simulink model "HILModel_flightgear"  (Simulink 7.8)
settings: Solver=ode4  StartTime=0.0  StopTime=inf  FixedStep=SampleT  RelTol=1e-3
InitFcn:
  | clc
  | hilInit
  | launchFlightgear
values from neighbouring files (symbols this model uses):
  Euler_0 = [0; 0*pi/180; 0*pi/180]'    [hilInit.m]
  HIL_K = 3    [hilInit.m]
  Pos_0 = [0; 0; 150]'    [hilInit.m]
  SampleT = 0.005    [hilInit.m]
  Vb_0 = [ 17; 0; 0]'    [hilInit.m]
  windBase = 3.5    [hilInit.m]
undefined symbols (not defined in the file or in its folder): A1, Apolar, barAdjust, baroOffset, baroScale, barTGain2, barTMean2, bPWMda, bPWMde, bPWMdr, bPWMdt, CD0, chord, CL0, CLa, CLa_dot, Clb, ClDa, CLDe, CLDf, ClDr, clock, Clp, CLq, Clr, Cm0, Cma, CmDe, CmDf, Cmq, Cnb, CnDa, CnDr, Cnp, Cnr, cubeAccelGain16405, cubeGyroGain16405, cubeMagGain16405, CYb, CYDr, da_failamp, da_failbias, da_failper, daL_fail, daR_fail, DiscIntNeverNeededParam, dr_fail, Earth, elarm, F, GS_location, ISA_g, Ixx, Iyy, Izz, Light, mass, MIL, MinThK, mPWMda ... (+14)
libraries: simulink x30, aerolibconvert2 x11, xpclib x8, aerolibactuator x5, aerolibwind2 x2, dspmtrx3 x2, aerolibfltsims x2, aerolibtransform2 x1, aerolibobsolete x1, aerolibatmos2 x1, aerolibanimutils x1
(part 1 of 3)
CloseFcn:
  | rtwprivate ssgencode ModelCloseRequest AttitudeComplementary
settings Model: Creator=ASL_Lab  LastModifiedBy=dagoodma
settings OptimizationCC: InitFltsAndDblsToZero=on
settings DebuggingCC: AlgebraicLoopMsg=error  SaveWithParameterizedLinksMsg=none  MultiTaskDSMMsg=warning  MultiTaskCondExecSysMsg=none  FcnCallInpInsideContextMsg=Use local settings  StrictBusMsg=None
settings HardwareCC: TargetHWDeviceType=32-bit Generic
settings SFSimCC: SimParseCustomCode=off
settings RTWCC: IncludeERTFirstTime=on
settings GRTTargetCC: TargetFcnLib=ansi_tfl_tmw.mat

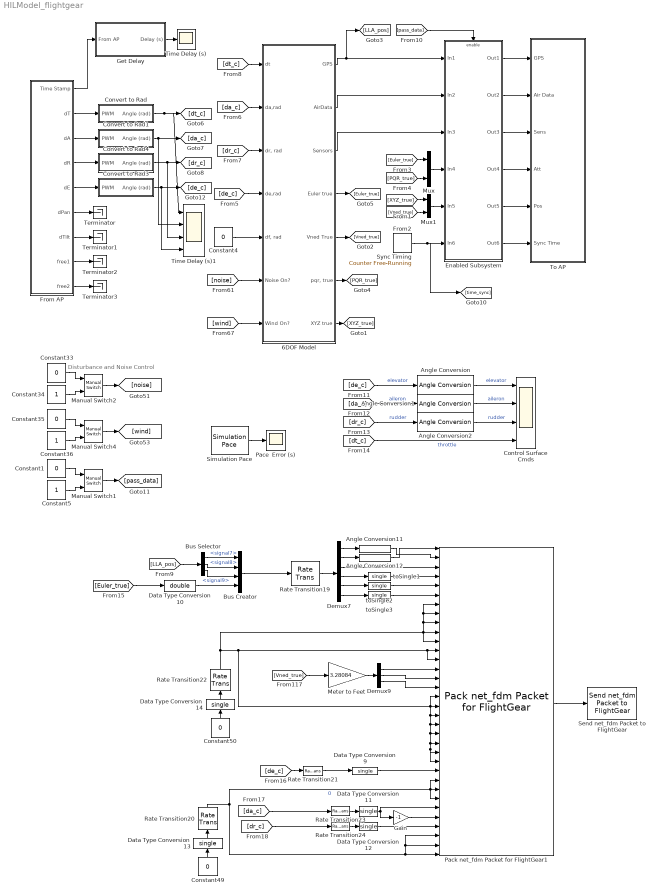
== system HILModel_flightgear ==
  note: Disturbance and Noise Control
  6DOF Model : Subsystem
  Angle Conversion : aerolibconvert2/Angle Conversion  IU=rad  OU=deg
  Angle Conversion1 : aerolibconvert2/Angle Conversion  IU=rad  OU=deg
  Angle Conversion11 : aerolibconvert2/Angle Conversion  IU=deg  OU=rad
  Angle Conversion12 : aerolibconvert2/Angle Conversion  IU=deg  OU=rad
  Angle Conversion2 : aerolibconvert2/Angle Conversion  IU=rad  OU=deg
  Bus Creator : BusCreator
  Bus Selector : BusSelector  OutputSignals=signal7,signal8,signal9
  Constant1 : Constant  Value=0  SampleTime=SampleT
  Constant33 : Constant  Value=0  SampleTime=SampleT
  Constant34 : Constant  SampleTime=SampleT
  Constant35 : Constant  Value=0  SampleTime=SampleT
  Constant36 : Constant  SampleTime=SampleT
  Constant4 : Constant  Value=0
  Constant49 : Constant  Value=0
  Constant5 : Constant  SampleTime=SampleT
  Constant50 : Constant  Value=0
  Control Surface Cmds : Scope  NumInputPorts=4
      settings: TimeRange=70  YMin=0.475~1.425~1.44~0.05  YMax=0.545~1.65~1.57~0.55  MaxDataPoints=25000
  Convert to Rad : Subsystem  mask{slopem=mPWMdt, interceptb=bPWMdt}
      mask prompts: slopem "Slope"; interceptb "Intercept"
  Convert to Rad1 : Subsystem  mask{slopem=mPWMda, interceptb=bPWMda}
      mask prompts: slopem "Slope"; interceptb "Intercept"
  Convert to Rad3 : Subsystem  mask{slopem=mPWMde, interceptb=bPWMde}
      mask prompts: slopem "Slope"; interceptb "Intercept"
  Convert to Rad4 : Subsystem  mask{slopem=mPWMdr, interceptb=bPWMdr}
      mask prompts: slopem "Slope"; interceptb "Intercept"
  Data Type Conversion10 : DataTypeConversion  OutDataTypeStr=double
  Data Type Conversion{9,11..14} (5 alike) : DataTypeConversion  OutDataTypeStr=single
  Demux7 : Demux  Outputs=6
  Demux9 : Demux  Outputs=3
  Enabled Subsystem : Subsystem  TreatAsAtomicUnit=on
  From AP : Subsystem
  Gain : Gain  Gain=-1
  Get Delay : Subsystem
  Manual Switch1 : simulink/Signal Routing/Manual Switch  sw=0  action=0  varsize=off
  Manual Switch2 : simulink/Signal Routing/Manual Switch  sw=1  action=0  varsize=off
  Manual Switch4 : simulink/Signal Routing/Manual Switch  sw=1  action=0  varsize=off
  Meter to Feet : Gain  Gain=3.28084
  Mux : Mux  Inputs=2
  Mux1 : Mux  Inputs=2
  Pace  Error (s) : Scope
      settings: YMin=-0.01  YMax=0.015  MaxDataPoints=25000
  Pack net_fdm Packet for FlightGear1 : aerolibfltsims/Pack net_fdm Packet for FlightGear  FlightGearVersion=v2.0  ShowPositionAttitudeInputs=on  ShowVelocityAccelerationInputs=on  ShowControlSurfacePositionInputs=on  ShowEngineFuelInputs=off  ShowLandingGearInputs=off  ShowEnvironmentInputs=off  SampleTime=SampleT
  Rate Transition{19,21,23..24} (4 alike) : RateTransition  Integrity=off  Deterministic=off  OutPortSampleTime=SampleT
  Rate Transition20 : RateTransition  OutPortSampleTime=SampleT
  Rate Transition22 : RateTransition  OutPortSampleTime=SampleT
  Send net_fdm Packet to FlightGear : aerolibfltsims/Send net_fdm Packet to FlightGear  DestinationIpAddress=127.0.0.1  DestinationPort=FLIGHTGEAR_UDP_FDM_PORT  LocalIpPort=-1  varLen=off  SampleTime=SampleT
  Simulation Pace : aerolibanimutils/Simulation Pace  SimulationPace=1  SleepMode=MATLAB Thread  OutputPaceError=on  SampleTime=SampleT
      settings: AttributesFormatString=%<SimulationPace> sec/sec
  Sync Timing : simulink/Sources/Counter Free-Running  NumBits=32  tsamp=SampleT
  Terminator{,1..3} (4 alike) : Terminator
  Time Delay (s) : Scope
      settings: TimeRange=60  YMin=0  YMax=0.05  SaveName=ScopeData2
  Time Delay (s)1 : Scope  NumInputPorts=4
      settings: TimeRange=60  YMin=-2.49294~0.78707~1.28363~-0.624215  YMax=-2.49294~0.78707~1.28363~-0.624215  SaveName=ScopeData3
  To AP : Subsystem
  toSingle1 : DataTypeConversion  OutDataTypeStr=single
  toSingle2 : DataTypeConversion  OutDataTypeStr=single
  toSingle3 : DataTypeConversion  OutDataTypeStr=single
  wires:
  [PQR_true] -> Mux/2
  [XYZ_true] -> Mux1/1
  [Vned_true] -> Mux1/2
  [Euler_true] -> Mux/1
  Enabled Subsystem/1(Out1) -> To AP/1(GPS)
  Enabled Subsystem/2(Out2) -> To AP/2(Air Data)
  Enabled Subsystem/3(Out3) -> To AP/3(Sens)
  Enabled Subsystem/4(Out4) -> To AP/4(Att)
  Enabled Subsystem/5(Out5) -> To AP/5(Pos)
  Enabled Subsystem/6(Out6) -> To AP/6(Sync Time)
  6DOF Model/1(GPS) -> Enabled Subsystem/1(In1), [LLA_pos]
  6DOF Model/2(AirData) -> Enabled Subsystem/2(In2)
  6DOF Model/3(Sensors) -> Enabled Subsystem/3(In3)
  Mux/1 -> Enabled Subsystem/4(In4)
  Mux1/1 -> Enabled Subsystem/5(In5)
  Sync Timing/1 -> Enabled Subsystem/6(In6), [time_sync]
  6DOF Model/4(Euler true) -> [Euler_true]
  6DOF Model/5(Vned True) -> [Vned_true]
  6DOF Model/6("pqr, true") -> [PQR_true]
  6DOF Model/7(XYZ true) -> [XYZ_true]
  Constant4/1 -> 6DOF Model/5("df, rad")
  Constant33/1 -> Manual Switch2/1
  Constant34/1 -> Manual Switch2/2
  Manual Switch2/1 -> [noise]
  Constant35/1 -> Manual Switch4/1
  Constant36/1 -> Manual Switch4/2
  Manual Switch4/1 -> [wind]
  [noise] -> 6DOF Model/6(Noise On?)
  [wind] -> 6DOF Model/7(Wind On?)
  Constant1/1 -> Manual Switch1/1
  Constant5/1 -> Manual Switch1/2
  Manual Switch1/1 -> [pass_data]
  [pass_data] -> Enabled Subsystem/Enable
  From AP/3(dA) -> Convert to Rad1/1(PWM)
  From AP/5(dE) -> Convert to Rad3/1(PWM)
  From AP/2(dT) -> Convert to Rad/1(PWM)
  From AP/4(dR) -> Convert to Rad4/1(PWM)
  Get Delay/1(Delay (s)) -> Time Delay (s)/1
  From AP/1(Time Stamp) -> Get Delay/1(From AP)
  Convert to Rad/1(Angle (rad)) -> [dt_c], Time Delay (s)1/1
  Convert to Rad1/1(Angle (rad)) -> [da_c], Time Delay (s)1/2
  From AP/6(dPan) -> Terminator/1
  [de_c] -> Angle Conversion/1  "elevator"
  [da_c] -> Angle Conversion1/1  "aileron"
  [dr_c] -> Angle Conversion2/1  "rudder"
  [dt_c] -> Control Surface Cmds/4  "throttle"
  [de_c] -> 6DOF Model/4(de,rad)
  [dt_c] -> 6DOF Model/1(dt)
  [dr_c] -> 6DOF Model/3("dr, rad")
  [da_c] -> 6DOF Model/2(da,rad)
  Angle Conversion/1 -> Control Surface Cmds/1  "elevator"
  Angle Conversion1/1 -> Control Surface Cmds/2  "aileron"
  Angle Conversion2/1 -> Control Surface Cmds/3  "rudder"
  Simulation Pace/1 -> Pace  Error (s)/1
  Convert to Rad4/1(Angle (rad)) -> [dr_c], Time Delay (s)1/3
  Convert to Rad3/1(Angle (rad)) -> [de_c], Time Delay (s)1/4
  From AP/7(dTilt) -> Terminator1/1
  From AP/8(free1) -> Terminator2/1
  From AP/9(free2) -> Terminator3/1
  Rate Transition19/1 -> Demux7/1
  Demux7/1 -> Angle Conversion11/1
  Demux7/2 -> Angle Conversion12/1
  Demux7/3 -> Pack net_fdm Packet for FlightGear1/3
  Demux7/4 -> toSingle1/1
  Demux7/5 -> toSingle2/1
  Demux7/6 -> toSingle3/1
  toSingle1/1 -> Pack net_fdm Packet for FlightGear1/4
  toSingle2/1 -> Pack net_fdm Packet for FlightGear1/5
  toSingle3/1 -> Pack net_fdm Packet for FlightGear1/6
  Pack net_fdm Packet for FlightGear1/1 -> Send net_fdm Packet to FlightGear/1
  Data Type Conversion12/1 -> Pack net_fdm Packet for FlightGear1/31
  Rate Transition20/1 -> Pack net_fdm Packet for FlightGear1/34, Pack net_fdm Packet for FlightGear1/33, Pack net_fdm Packet for FlightGear1/32, Pack net_fdm Packet for FlightGear1/26, Pack net_fdm Packet for FlightGear1/27, Pack net_fdm Packet for FlightGear1/28  "0"
  Rate Transition21/1 -> Data Type Conversion9/1
  Rate Transition23/1 -> Data Type Conversion11/1
  Data Type Conversion13/1 -> Rate Transition20/1
  Constant49/1 -> Data Type Conversion13/1
  Rate Transition24/1 -> Data Type Conversion12/1
  Data Type Conversion11/1 -> Gain/1, Pack net_fdm Packet for FlightGear1/29
  Gain/1 -> Pack net_fdm Packet for FlightGear1/30
  Angle Conversion12/1 -> Pack net_fdm Packet for FlightGear1/1
  Angle Conversion11/1 -> Pack net_fdm Packet for FlightGear1/2
  Data Type Conversion9/1 -> Pack net_fdm Packet for FlightGear1/25
  Data Type Conversion14/1 -> Rate Transition22/1
  Constant50/1 -> Data Type Conversion14/1
  Rate Transition22/1 -> Pack net_fdm Packet for FlightGear1/10, Pack net_fdm Packet for FlightGear1/11, Pack net_fdm Packet for FlightGear1/9, Pack net_fdm Packet for FlightGear1/7, Pack net_fdm Packet for FlightGear1/8, Pack net_fdm Packet for FlightGear1/12, Pack net_fdm Packet for FlightGear1/13, Pack net_fdm Packet for FlightGear1/18, Pack net_fdm Packet for FlightGear1/17, Pack net_fdm Packet for FlightGear1/19, Pack net_fdm Packet for FlightGear1/20, Pack net_fdm Packet for FlightGear1/21, Pack net_fdm Packet for FlightGear1/22, Pack net_fdm Packet for FlightGear1/23, Pack net_fdm Packet for FlightGear1/24
  Demux9/1 -> Pack net_fdm Packet for FlightGear1/14
  Demux9/3 -> Pack net_fdm Packet for FlightGear1/16
  Demux9/2 -> Pack net_fdm Packet for FlightGear1/15
  [Vned_true] -> Meter to Feet/1
  Meter to Feet/1 -> Demux9/1
  [Euler_true] -> Data Type Conversion10/1
  [LLA_pos] -> Bus Selector/1
  Bus Selector/1 -> Bus Creator/1  "<signal7>"
  Bus Selector/2 -> Bus Creator/2  "<signal8>"
  Bus Selector/3 -> Bus Creator/3  "<signal9>"
  Data Type Conversion10/1 -> Bus Creator/4
  Bus Creator/1 -> Rate Transition19/1
  [de_c] -> Rate Transition21/1
  [da_c] -> Rate Transition23/1
  [dr_c] -> Rate Transition24/1

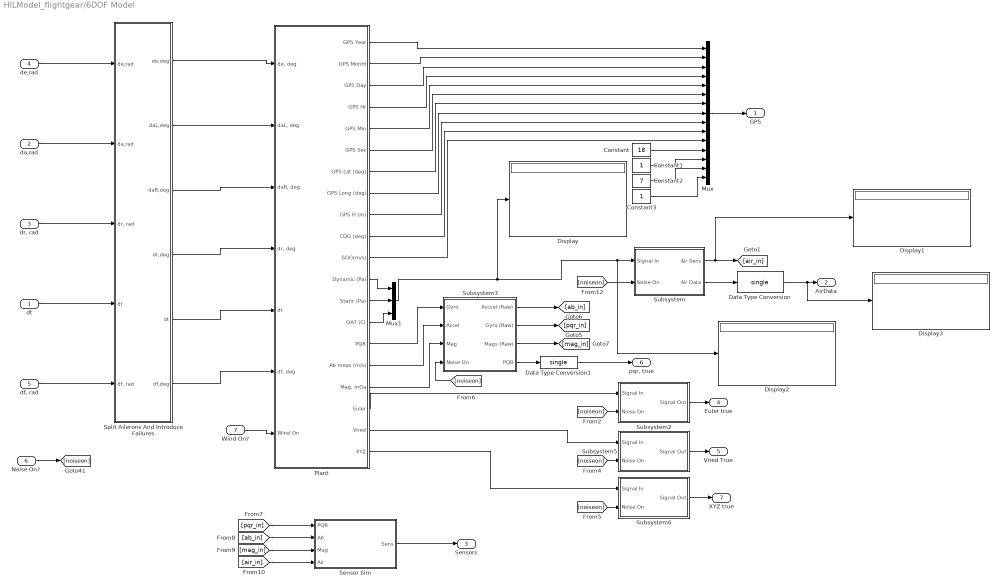
== system HILModel_flightgear/6DOF Model ==
  dt : Inport
  da,rad : Inport  Port=2
  "dr, rad" : Inport  Port=3
  de,rad : Inport  Port=4
  "df, rad" : Inport  Port=5
  Noise On? : Inport  Port=6
  Wind On? : Inport  Port=7
  Constant : Constant  Value=18  SampleTime=SampleT
  Constant1 : Constant  SampleTime=SampleT
  Constant2 : Constant  Value=7  SampleTime=SampleT
  Constant3 : Constant  SampleTime=SampleT
  Data Type Conversion : DataTypeConversion  OutDataTypeStr=single
  Data Type Conversion1 : DataTypeConversion  OutDataTypeStr=single
  Display{,1..3} (4 alike) : Display
  Mux : Mux  Inputs=15
  Mux1 : Mux  Inputs=3
  Plant : Subsystem
  Sensor Sim : Subsystem
  Split Ailerons And Introduce Failures : Subsystem
  Subsystem : Subsystem  mask{nv=[0.01 0.01 0.1], st=SampleT, ns=[132 564 987]}
      mask prompts: nv "Noise Variance"; st "Sample Time"; ns "Noise Seed"
  Subsystem2 : Subsystem  mask{nv=[0.0001 0.00003 0.0001], st=SampleT, ns=[132 564 987]}
      mask prompts: nv "Noise Variance"; st "Sample Time"; ns "Noise Seed"
  Subsystem3 : Subsystem  mask{accelVar=[0.1 0.1 0.1], accelSeed=[132 564 987], hilCubeAccelGain=cubeAccelGain16405, gyroVar=[0.1 0.1 0.1], gyroSeed=[132 564 987], hilCubeGyroGain=cubeGyroGain16405, magVar=[0.1 0.1 0.1], magSeed=[132 564 987], hilCubeMagGain=cubeMagGain16405, st=SampleT}
      mask prompts: accelVar "Accelerometer Noise Variance"; accelSeed "Accelerometer Noise Seed"; hilCubeAccelGain "Accelerometer Gain"; gyroVar "Gyro Noise Variance"; gyroSeed "Gyro Noise Seed"; hilCubeGyroGain "Gyro Gain"; magVar "Magnetometer Noise Variance"; magSeed "Magnetometer Noise Seed"; hilCubeMagGain "Magnetometer Gain"; st "Sample Time"
  Subsystem5 : Subsystem  mask{nv=[0.01 0.01 0.01], st=SampleT, ns=[321564 6546 98798]}
      mask prompts: nv "Noise Variance"; st "Sample Time"; ns "Noise Seed"
  Subsystem6 : Subsystem  mask{nv=[0.05 0.05 0.07], st=SampleT, ns=[321564]}
      mask prompts: nv "Noise Variance"; st "Sample Time"; ns "Noise Seed"
  GPS : Outport
  AirData : Outport  Port=2
  Sensors : Outport  Port=3
  Euler true : Outport  Port=4
  Vned True : Outport  Port=5
  "pqr, true" : Outport  Port=6
  XYZ true : Outport  Port=7
  wires:
  Data Type Conversion/1 -> AirData/1, Display3/1
  Wind On?/1 -> Plant/7(Wind On)
  Plant/20(XYZ) -> Subsystem6/1(Signal In)
  Subsystem6/1(Signal Out) -> XYZ true/1
  Plant/19(Vned) -> Subsystem5/1(Signal In)
  Subsystem5/1(Signal Out) -> Vned True/1
  Plant/18(Euler) -> Subsystem2/1(Signal In)
  Subsystem2/1(Signal Out) -> Euler true/1
  [noiseon] -> Subsystem3/4(Noise On)
  [noiseon] -> Subsystem6/2(Noise On)
  [noiseon] -> Subsystem5/2(Noise On)
  [noiseon] -> Subsystem2/2(Noise On)
  [noiseon] -> Subsystem/2(Noise On)
  Subsystem/1(Air Sens) -> [air_in], Display1/1
  Noise On?/1 -> [noiseon]
  Constant3/1 -> Mux/15
  Constant2/1 -> Mux/14
  Constant1/1 -> Mux/13
  Constant/1 -> Mux/12
  Mux1/1 -> Subsystem/1(Signal In), Display2/1, Display/1
  Plant/14(OAT (C)) -> Mux1/3
  Plant/13(Static (Pa)) -> Mux1/2
  Plant/11(SOG(m/s)) -> Mux/11
  Plant/10(COG (deg)) -> Mux/10
  Plant/9(GPS H (m)) -> Mux/9
  Plant/8(GPS Long (deg)) -> Mux/8
  Plant/7(GPS Lat (deg)) -> Mux/7
  Plant/6(GPS Sec) -> Mux/6
  Plant/5(GPS Min) -> Mux/5
  Plant/4(GPS Hr) -> Mux/4
  Plant/3(GPS Day) -> Mux/3
  Plant/2(GPS Month) -> Mux/2
  Plant/1(GPS Year) -> Mux/1
  Mux/1 -> GPS/1
  "df, rad"/1 -> Split Ailerons And Introduce Failures/5("df, rad")
  dt/1 -> Split Ailerons And Introduce Failures/4(dt)
  "dr, rad"/1 -> Split Ailerons And Introduce Failures/3("dr, rad")
  da,rad/1 -> Split Ailerons And Introduce Failures/2(da,rad)
  de,rad/1 -> Split Ailerons And Introduce Failures/1(de,rad)
  [pqr_in] -> Sensor Sim/1(PQR)
  [ab_in] -> Sensor Sim/2(Ab)
  [mag_in] -> Sensor Sim/3(Mag)
  Split Ailerons And Introduce Failures/1(de,deg) -> Plant/1("de, deg")
  Split Ailerons And Introduce Failures/2(daL,deg) -> Plant/2("daL, deg")
  Split Ailerons And Introduce Failures/3(daR,deg) -> Plant/3("daR, deg")
  Split Ailerons And Introduce Failures/4(dr,deg) -> Plant/4("dr, deg")
  Split Ailerons And Introduce Failures/5("dt ") -> Plant/5(dt)
  Split Ailerons And Introduce Failures/6(df,deg) -> Plant/6("df, deg")
  [air_in] -> Sensor Sim/4(Air)
  Plant/15(PQR) -> Subsystem3/1(Gyro)
  Plant/16(Ab meas (m/s)) -> Subsystem3/2(Accel)
  Plant/17("Mag, mGa") -> Subsystem3/3(Mag)
  Subsystem3/4("PQR ") -> Data Type Conversion1/1
  Subsystem3/1(Acccel (Raw)) -> [ab_in]
  Subsystem3/2("Gyro (Raw)  ") -> [pqr_in]
  Subsystem3/3(Mags (Raw)) -> [mag_in]
  Sensor Sim/1(Sens) -> Sensors/1
  Data Type Conversion1/1 -> "pqr, true"/1
  Subsystem/2(Air Data) -> Data Type Conversion/1
  Plant/12(Dynamic (Pa)) -> Mux1/1

== system HILModel_flightgear/Convert to Rad ==
  PWM : Inport
  Add : Sum
  Constant1 : Constant  Value=slopem
  Constant2 : Constant  Value=interceptb
  Data Type Conversion : DataTypeConversion  OutDataTypeStr=single
  Divide : Product
  Angle (rad) : Outport
  wires:
  Constant1/1 -> Divide/2
  Add/1 -> Data Type Conversion/1
  Divide/1 -> Add/1
  Constant2/1 -> Add/2
  PWM/1 -> Divide/1
  Data Type Conversion/1 -> Angle (rad)/1

== system HILModel_flightgear/Convert to Rad1 ==
  PWM : Inport
  Add : Sum
  Constant1 : Constant  Value=slopem
  Constant2 : Constant  Value=interceptb
  Data Type Conversion : DataTypeConversion  OutDataTypeStr=single
  Divide : Product
  Angle (rad) : Outport
  wires:
  Data Type Conversion/1 -> Angle (rad)/1
  PWM/1 -> Divide/1
  Constant2/1 -> Add/2
  Divide/1 -> Add/1
  Add/1 -> Data Type Conversion/1
  Constant1/1 -> Divide/2

== system HILModel_flightgear/Convert to Rad3 ==
  PWM : Inport
  Add : Sum
  Constant1 : Constant  Value=slopem
  Constant2 : Constant  Value=interceptb
  Data Type Conversion : DataTypeConversion  OutDataTypeStr=single
  Divide : Product
  Angle (rad) : Outport
  wires:
  Data Type Conversion/1 -> Angle (rad)/1
  PWM/1 -> Divide/1
  Constant2/1 -> Add/2
  Divide/1 -> Add/1
  Add/1 -> Data Type Conversion/1
  Constant1/1 -> Divide/2

== system HILModel_flightgear/Convert to Rad4 ==
  PWM : Inport
  Add : Sum
  Constant1 : Constant  Value=slopem
  Constant2 : Constant  Value=interceptb
  Data Type Conversion : DataTypeConversion  OutDataTypeStr=single
  Divide : Product
  Angle (rad) : Outport
  wires:
  Data Type Conversion/1 -> Angle (rad)/1
  PWM/1 -> Divide/1
  Constant2/1 -> Add/2
  Divide/1 -> Add/1
  Add/1 -> Data Type Conversion/1
  Constant1/1 -> Divide/2

== system HILModel_flightgear/Enabled Subsystem ==
  In1 : Inport
  In2 : Inport  Port=2
  In3 : Inport  Port=3
  In4 : Inport  Port=4
  In5 : Inport  Port=5
  In6 : Inport  Port=6
  Enable : EnablePort
  Out1 : Outport
  Out2 : Outport  Port=2
  Out3 : Outport  Port=3
  Out4 : Outport  Port=4
  Out5 : Outport  Port=5
  Out6 : Outport  Port=6
  wires:
  In1/1 -> Out1/1
  In2/1 -> Out2/1
  In3/1 -> Out3/1
  In4/1 -> Out4/1
  In5/1 -> Out5/1
  In6/1 -> Out6/1

== system HILModel_flightgear/From AP ==
  Display{,1..4} (5 alike) : Display
  Receive : xpclib/UDP/Receive  ipAddress=0.0.0.0  ipPort=5678  width=20  vblLen=off  sampletime=SampleT
  Subsystem : Subsystem
  Subsystem1 : Subsystem
  Subsystem2 : Subsystem
  Subsystem3 : Subsystem
  Terminator : Terminator
  Unpack1 : xpclib/UDP/Unpack  dimensions={1,1,1,1,1,1,1,1,1}  datatypes={'uint16','uint16','uint16','uint16', 'uint16', 'uint16','uint16', 'uint16','uint32'}  byteAlign=1
  Time Stamp : Outport
  dT : Outport  Port=2
  dA : Outport  Port=3
  dR : Outport  Port=4
  dE : Outport  Port=5
  dPan : Outport  Port=6
  dTilt : Outport  Port=7
  free1 : Outport  Port=8
  free2 : Outport  Port=9
  wires:
  Receive/1 -> Unpack1/1
  Receive/2 -> Terminator/1
  Unpack1/1 -> Subsystem/1(uS)  "dt"
  Unpack1/3 -> Subsystem2/1(uS)  "dr"
  Unpack1/5 -> dPan/1  "dpan"
  Unpack1/7 -> free1/1  "free1"
  Unpack1/9 -> Time Stamp/1, Display4/1  "timeStamp"
  Unpack1/2 -> Subsystem1/1(uS)  "da"
  Unpack1/4 -> Subsystem3/1(uS)  "de"
  Unpack1/6 -> dTilt/1  "dtilt"
  Unpack1/8 -> free2/1  "free2"
  Subsystem/1(PWM) -> dT/1, Display/1
  Subsystem1/1(PWM) -> dA/1, Display1/1
  Subsystem2/1(PWM) -> dR/1, Display2/1
  Subsystem3/1(PWM) -> dE/1, Display3/1

== system HILModel_flightgear/Get Delay ==
  From AP : Inport
  Detect Change : Subsystem
  GPSAlive : Subsystem
  Delay (s) : Outport
  wires:
  From AP/1 -> Detect Change/1(Data)
  Detect Change/1(change?) -> GPSAlive/1(update?)
  GPSAlive/1(Update TIme) -> Delay (s)/1

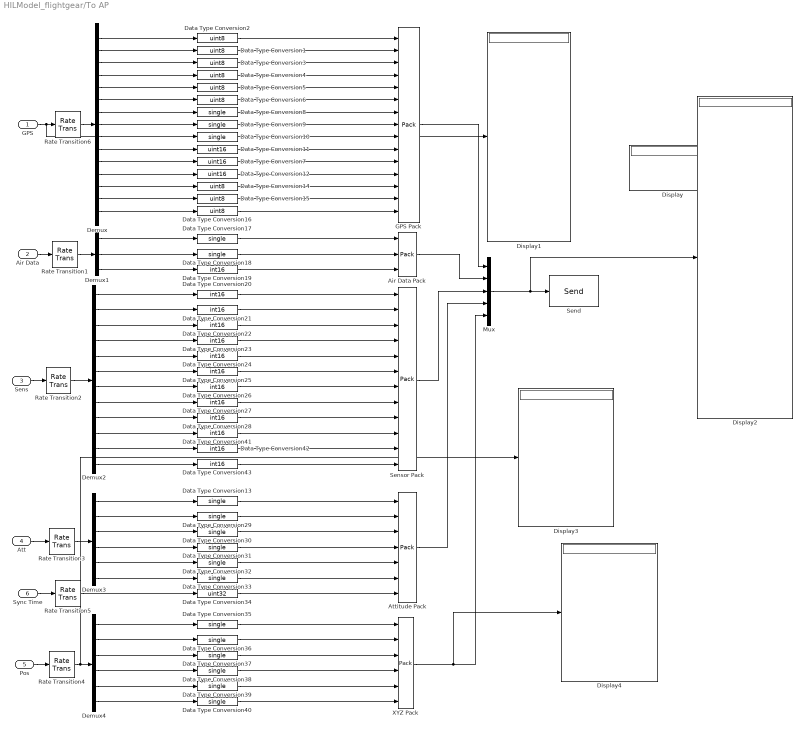
== system HILModel_flightgear/To AP ==
  GPS : Inport
  Air Data : Inport  Port=2
  Sens : Inport  Port=3
  Att : Inport  Port=4
  Pos : Inport  Port=5
  Sync Time : Inport  Port=6
  Air Data Pack : xpclib/UDP/Pack  datatypes={'single', 'single', 'int16'}  byteAlign=1
  Attitude Pack : xpclib/UDP/Pack  datatypes={'single','single','single','single','single','single','uint32'}  byteAlign=1
  Data Type Conversion{1..6,14..16} (9 alike) : DataTypeConversion  OutDataTypeStr=uint8
  Data Type Conversion{8..10,13,17..18,29..33,35..40} (17 alike) : DataTypeConversion  OutDataTypeStr=single
  Data Type Conversion11 : DataTypeConversion  OutDataTypeStr=uint16
  Data Type Conversion12 : DataTypeConversion  OutDataTypeStr=uint16
  Data Type Conversion{19..28,41..43} (13 alike) : DataTypeConversion  OutDataTypeStr=int16
  Data Type Conversion34 : DataTypeConversion  OutDataTypeStr=uint32
  Data Type Conversion7 : DataTypeConversion  OutDataTypeStr=uint16
  Demux : Demux  Outputs=15
  Demux1 : Demux  Outputs=3
  Demux2 : Demux  Outputs=12
  Demux3 : Demux  Outputs=6
  Demux4 : Demux  Outputs=6
  Display{,1..4} (5 alike) : Display
  GPS Pack : xpclib/UDP/Pack  datatypes={'uint8','uint8','uint8','uint8','uint8','uint8', 'single', 'single', 'single', 'uint16', 'uint16', 'uint16', 'uint8', 'uint8', 'uint8'}  byteAlign=1
  Mux : Mux  Inputs=5
  Rate Transition{1..6} (6 alike) : RateTransition  OutPortSampleTime=SampleT*HIL_K
  Send : xpclib/UDP/Send  ipAddress=255.255.255.255  ipPort=5679  localPort=5678  vblLen=off  sampletime=SampleT*HIL_K
  Sensor Pack : xpclib/UDP/Pack  datatypes={'int16', 'int16', 'int16', 'int16', 'int16', 'int16', 'int16', 'int16', 'int16', 'int16', 'int16', 'int16'}  byteAlign=1
  XYZ Pack : xpclib/UDP/Pack  datatypes={'single','single','single','single','single','single'}  byteAlign=1
  wires:
  Demux/1 -> Data Type Conversion2/1
  Demux/2 -> Data Type Conversion1/1
  Demux/3 -> Data Type Conversion3/1
  Demux/4 -> Data Type Conversion4/1
  Demux/5 -> Data Type Conversion5/1
  Demux/6 -> Data Type Conversion6/1
  Demux/7 -> Data Type Conversion8/1
  Demux/8 -> Data Type Conversion9/1
  Demux/9 -> Data Type Conversion10/1
  Demux/10 -> Data Type Conversion11/1
  Demux/11 -> Data Type Conversion7/1
  Demux/12 -> Data Type Conversion12/1
  Demux/13 -> Data Type Conversion14/1
  Demux/14 -> Data Type Conversion15/1
  Demux/15 -> Data Type Conversion16/1
  Demux1/2 -> Data Type Conversion18/1
  Demux1/3 -> Data Type Conversion19/1
  Demux2/1 -> Data Type Conversion20/1
  Demux2/2 -> Data Type Conversion21/1
  Demux2/3 -> Data Type Conversion22/1
  Demux2/4 -> Data Type Conversion23/1
  Demux2/5 -> Data Type Conversion24/1
  Demux2/6 -> Data Type Conversion25/1
  Demux2/7 -> Data Type Conversion26/1
  Demux2/8 -> Data Type Conversion27/1
  Demux2/9 -> Data Type Conversion28/1
  Mux/1 -> Send/1, Display2/1
  GPS Pack/1 -> Mux/1
  Air Data Pack/1 -> Mux/2
  Sensor Pack/1 -> Mux/3
  GPS/1 -> Rate Transition6/1, Display1/1
  Air Data/1 -> Rate Transition1/1
  Sens/1 -> Rate Transition2/1
  Rate Transition6/1 -> Demux/1
  Rate Transition1/1 -> Demux1/1
  Rate Transition2/1 -> Demux2/1
  Att/1 -> Rate Transition3/1
  Pos/1 -> Rate Transition4/1
  Rate Transition3/1 -> Demux3/1
  Demux3/1 -> Data Type Conversion13/1
  Demux3/2 -> Data Type Conversion29/1
  Demux3/3 -> Data Type Conversion30/1
  Demux3/4 -> Data Type Conversion31/1
  Demux3/5 -> Data Type Conversion32/1
  Demux3/6 -> Data Type Conversion33/1
  Demux4/1 -> Data Type Conversion35/1
  Demux4/2 -> Data Type Conversion36/1
  Demux4/3 -> Data Type Conversion37/1
  Demux4/4 -> Data Type Conversion38/1
  Demux4/5 -> Data Type Conversion39/1
  Demux4/6 -> Data Type Conversion40/1
  Rate Transition4/1 -> Demux4/1, Display3/1
  Attitude Pack/1 -> Mux/4
  XYZ Pack/1 -> Mux/5, Display4/1
  Sync Time/1 -> Rate Transition5/1
  Data Type Conversion2/1 -> GPS Pack/1
  Data Type Conversion1/1 -> GPS Pack/2
  Data Type Conversion3/1 -> GPS Pack/3
  Data Type Conversion4/1 -> GPS Pack/4
  Data Type Conversion5/1 -> GPS Pack/5
  Data Type Conversion6/1 -> GPS Pack/6
  Data Type Conversion8/1 -> GPS Pack/7
  Data Type Conversion9/1 -> GPS Pack/8
  Data Type Conversion10/1 -> GPS Pack/9
  Data Type Conversion11/1 -> GPS Pack/10
  Data Type Conversion7/1 -> GPS Pack/11
  Data Type Conversion12/1 -> GPS Pack/12
  Data Type Conversion14/1 -> GPS Pack/13
  Data Type Conversion15/1 -> GPS Pack/14
  Data Type Conversion16/1 -> GPS Pack/15
  Data Type Conversion17/1 -> Air Data Pack/1
  Data Type Conversion18/1 -> Air Data Pack/2
  Data Type Conversion19/1 -> Air Data Pack/3
  Data Type Conversion20/1 -> Sensor Pack/1
  Data Type Conversion21/1 -> Sensor Pack/2
  Data Type Conversion22/1 -> Sensor Pack/3
  Data Type Conversion23/1 -> Sensor Pack/4
  Data Type Conversion24/1 -> Sensor Pack/5
  Data Type Conversion25/1 -> Sensor Pack/6
  Data Type Conversion26/1 -> Sensor Pack/7
  Data Type Conversion27/1 -> Sensor Pack/8
  Data Type Conversion28/1 -> Sensor Pack/9
  Data Type Conversion13/1 -> Attitude Pack/1
  Data Type Conversion29/1 -> Attitude Pack/2
  Data Type Conversion30/1 -> Attitude Pack/3
  Data Type Conversion31/1 -> Attitude Pack/4
  Data Type Conversion32/1 -> Attitude Pack/5
  Data Type Conversion33/1 -> Attitude Pack/6
  Data Type Conversion34/1 -> Attitude Pack/7
  Data Type Conversion35/1 -> XYZ Pack/1
  Data Type Conversion36/1 -> XYZ Pack/2
  Data Type Conversion37/1 -> XYZ Pack/3
  Data Type Conversion38/1 -> XYZ Pack/4
  Data Type Conversion39/1 -> XYZ Pack/5
  Data Type Conversion40/1 -> XYZ Pack/6
  Demux1/1 -> Data Type Conversion17/1
  Rate Transition5/1 -> Data Type Conversion34/1
  Demux2/10 -> Data Type Conversion41/1
  Data Type Conversion41/1 -> Sensor Pack/10
  Demux2/11 -> Data Type Conversion42/1
  Data Type Conversion42/1 -> Sensor Pack/11
  Demux2/12 -> Data Type Conversion43/1
  Data Type Conversion43/1 -> Sensor Pack/12

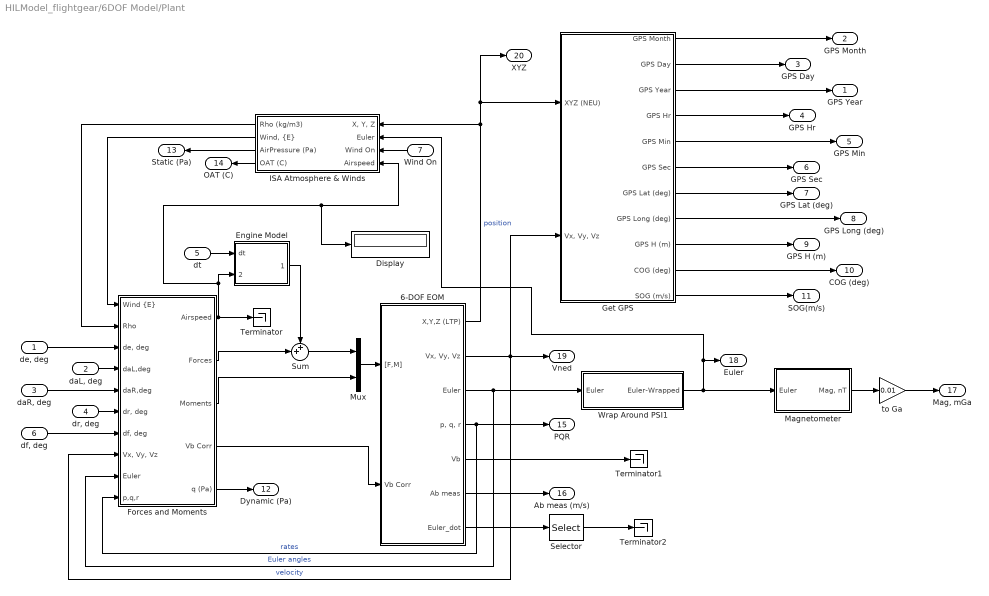
== system HILModel_flightgear/6DOF Model/Plant ==
  "de, deg" : Inport
  "daL, deg" : Inport  Port=2
  "daR, deg" : Inport  Port=3
  "dr, deg" : Inport  Port=4
  dt : Inport  Port=5
  "df, deg" : Inport  Port=6
  Wind On : Inport  Port=7
  6-DOF EOM : Subsystem
  Display : Display
  Engine Model : Subsystem
  Forces and Moments : Subsystem
  Get GPS : Subsystem
  ISA Atmosphere & Winds : Subsystem
  Magnetometer : Subsystem  mask{magField=[ 27590.4 1999.5 30223.2]}
      mask prompts: magField "Local Magnetic Field"
      mask help:
      | Simulates the Data from magnetometers with no noise.
      |
      | You can obtain data for the local magnetic field at:
      |
      | http://www.ngdc.noaa.gov/geomagmodels/IGRFWMM.jsp
  Mux : Mux  Inputs=2
  Selector : Selector  InputPortWidth=3  IndexOptions=Index vector (dialog)  Indices=[3]  OutputSizes=1
  Sum : Sum  Inputs=++|  SaturateOnIntegerOverflow=on
  Terminator : Terminator
  Terminator1 : Terminator
  Terminator2 : Terminator
  Wrap Around PSI1 : Subsystem
  to Ga : Gain  Gain=0.01
  GPS Year : Outport
  GPS Month : Outport  Port=2
  GPS Day : Outport  Port=3
  GPS Hr : Outport  Port=4
  GPS Min : Outport  Port=5
  GPS Sec : Outport  Port=6
  GPS Lat (deg) : Outport  Port=7
  GPS Long (deg) : Outport  Port=8
  GPS H (m) : Outport  Port=9
  COG (deg) : Outport  Port=10
  SOG(m/s) : Outport  Port=11
  Dynamic (Pa) : Outport  Port=12
  Static (Pa) : Outport  Port=13
  OAT (C) : Outport  Port=14
  PQR : Outport  Port=15
  Ab meas (m/s) : Outport  Port=16
  "Mag, mGa" : Outport  Port=17
  Euler : Outport  Port=18
  Vned : Outport  Port=19
  XYZ : Outport  Port=20
  wires:
  Get GPS/1(GPS Month) -> GPS Month/1
  Get GPS/2(GPS Day) -> GPS Day/1
  Get GPS/3(GPS Year) -> GPS Year/1
  Get GPS/4(GPS Hr) -> GPS Hr/1
  Get GPS/5(GPS Min) -> GPS Min/1
  Get GPS/6(GPS Sec) -> GPS Sec/1
  Get GPS/7(GPS Lat (deg)) -> GPS Lat (deg)/1
  Get GPS/8(GPS Long (deg)) -> GPS Long (deg)/1
  Get GPS/9(GPS H (m)) -> GPS H (m)/1
  6-DOF EOM/6(Ab meas) -> Ab meas (m/s)/1
  Mux/1 -> 6-DOF EOM/1("[F,M]")
  6-DOF EOM/5(Vb) -> Terminator1/1
  Engine Model/1(Thrust) -> Sum/1
  Forces and Moments/5(q (Pa)) -> Dynamic (Pa)/1
  ISA Atmosphere & Winds/3(AirPressure (Pa)) -> Static (Pa)/1
  Forces and Moments/1(Airspeed) -> Engine Model/2(Vmag), ISA Atmosphere & Winds/4(Airspeed), Display/1, Terminator/1
  ISA Atmosphere & Winds/2("Wind, {E}") -> Forces and Moments/1("Wind {E}")
  ISA Atmosphere & Winds/1(Rho (kg/m3)) -> Forces and Moments/2(Rho)
  Forces and Moments/3(Moments) -> Mux/2
  Forces and Moments/2(Forces) -> Sum/2
  Sum/1 -> Mux/1
  Forces and Moments/4(Vb Corr) -> 6-DOF EOM/2(Vb Corr)
  6-DOF EOM/1(X,Y,Z (LTP)) -> ISA Atmosphere & Winds/1("X, Y, Z"), Get GPS/1(XYZ (NEU)), XYZ/1  "position"
  6-DOF EOM/2("Vx, Vy, Vz") -> Vned/1, Get GPS/2("Vx, Vy, Vz"), Forces and Moments/8("Vx, Vy, Vz ")  "velocity"
  6-DOF EOM/3(Euler) -> Wrap Around PSI1/1(Euler), Forces and Moments/9(Euler)  "Euler angles"
  6-DOF EOM/4("p, q, r") -> PQR/1, Forces and Moments/10(p,q,r)  "rates"
  dt/1 -> Engine Model/1(dt)
  "de, deg"/1 -> Forces and Moments/3("de, deg")
  "daL, deg"/1 -> Forces and Moments/4(daL,deg)
  "dr, deg"/1 -> Forces and Moments/6("dr, deg")
  "df, deg"/1 -> Forces and Moments/7("df, deg")
  Wrap Around PSI1/1(Euler-Wrapped) -> Magnetometer/1(Euler), Euler/1, ISA Atmosphere & Winds/2(Euler)
  Magnetometer/1("Mag, nT") -> to Ga/1
  Get GPS/10(COG (deg)) -> COG (deg)/1
  Get GPS/11(SOG (m/s)) -> SOG(m/s)/1
  ISA Atmosphere & Winds/4(OAT (C)) -> OAT (C)/1
  6-DOF EOM/7(Euler_dot) -> Selector/1
  Selector/1 -> Terminator2/1
  Wind On/1 -> ISA Atmosphere & Winds/3(Wind On)
  "daR, deg"/1 -> Forces and Moments/5(daR,deg)
  to Ga/1 -> "Mag, mGa"/1

== system HILModel_flightgear/6DOF Model/Sensor Sim ==
  PQR : Inport
  Ab : Inport  Port=2
  Mag : Inport  Port=3
  Air : Inport  Port=4
  Mux2 : Mux
  Sens : Outport
  wires:
  Mux2/1 -> Sens/1
  Air/1 -> Mux2/4
  PQR/1 -> Mux2/1
  Ab/1 -> Mux2/2
  Mag/1 -> Mux2/3

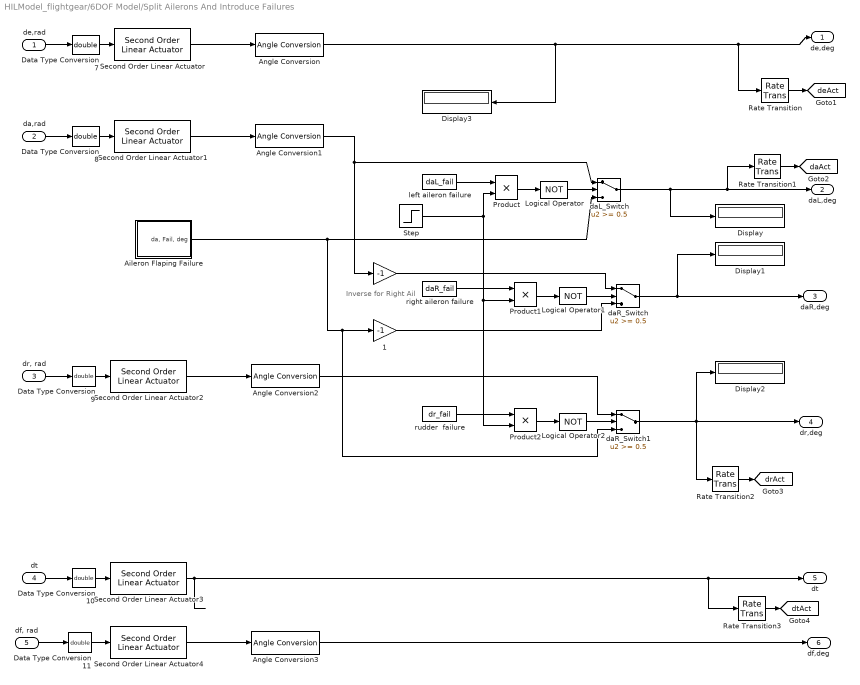
== system HILModel_flightgear/6DOF Model/Split Ailerons And Introduce Failures ==
  note: Inverse
      | for Right
      | Ail
  de,rad : Inport
  da,rad : Inport  Port=2
  "dr, rad" : Inport  Port=3
  dt : Inport  Port=4
  "df, rad" : Inport  Port=5
  " " : Gain  Gain=-1  SaturateOnIntegerOverflow=on  OutDataTypeStr=Inherit: Same as input  ParamDataTypeStr=Inherit: Same as input
  " 1" : Gain  Gain=-1  SaturateOnIntegerOverflow=on  OutDataTypeStr=Inherit: Same as input  ParamDataTypeStr=Inherit: Same as input
  Aileron Flaping Failure : Subsystem
  Angle Conversion{,1..3} (4 alike) : aerolibconvert2/Angle Conversion  IU=rad  OU=deg
  Data Type Conversion{7..11} (5 alike) : DataTypeConversion  OutDataTypeStr=double
  Display{,1..3} (4 alike) : Display
  Logical Operator : Logic  Operator=NOT  AllPortsSameDT=off  OutDataTypeStr=boolean
  Logical Operator1 : Logic  Operator=NOT  AllPortsSameDT=off  OutDataTypeStr=boolean
  Logical Operator2 : Logic  Operator=NOT  AllPortsSameDT=off  OutDataTypeStr=boolean
  Product : Product  RndMeth=Zero
  Product1 : Product  RndMeth=Zero
  Product2 : Product  RndMeth=Zero
  Rate Transition{,1..3} (4 alike) : RateTransition  OutPortSampleTime=apSampleTime
  Second Order Linear Actuator{,1..3} (4 alike) : aerolibactuator/Second Order Linear Actuator  wn_fin=15  z_fin=0.8  fin_act_0=0
  Second Order Linear Actuator4 : aerolibactuator/Second Order Linear Actuator  wn_fin=150  z_fin=0.7  fin_act_0=0
  Step : Step  Time=tfailure
  daL_Switch : Switch  Threshold=0.5
  daR_Switch : Switch  Threshold=0.5
  daR_Switch1 : Switch  Threshold=0.5
  left aileron failure : Constant  Value=daL_fail
  right aileron failure : Constant  Value=daR_fail
  rudder  failure : Constant  Value=dr_fail
  de,deg : Outport
  daL,deg : Outport  Port=2
  daR,deg : Outport  Port=3
  dr,deg : Outport  Port=4
  "dt " : Outport  Port=5
  df,deg : Outport  Port=6
  tag scope: daAct=global, deAct=global, drAct=global, dtAct=global
  wires:
  Rate Transition/1 -> [deAct]
  daR_Switch1/1 -> Rate Transition2/1, Display2/1, dr,deg/1
  Logical Operator2/1 -> daR_Switch1/2
  Product2/1 -> Logical Operator2/1
  rudder  failure/1 -> Product2/1
  daR_Switch/1 -> Display1/1, daR,deg/1
  " 1"/1 -> daR_Switch/3
  " "/1 -> daR_Switch/1
  Logical Operator1/1 -> daR_Switch/2
  Product1/1 -> Logical Operator1/1
  right aileron failure/1 -> Product1/1
  daL_Switch/1 -> Rate Transition1/1, daL,deg/1, Display/1
  Step/1 -> Product2/2, Product1/2, Product/2
  Logical Operator/1 -> daL_Switch/2
  Product/1 -> Logical Operator/1
  Aileron Flaping Failure/1("da, Fail, deg") -> daR_Switch1/3, " 1"/1, daL_Switch/3
  left aileron failure/1 -> Product/1
  Angle Conversion3/1 -> df,deg/1
  Angle Conversion2/1 -> daR_Switch1/1
  Angle Conversion1/1 -> " "/1, daL_Switch/1
  Angle Conversion/1 -> Rate Transition/1, de,deg/1, Display3/1
  Data Type Conversion11/1 -> Second Order Linear Actuator4/1
  Data Type Conversion10/1 -> Second Order Linear Actuator3/1
  Data Type Conversion9/1 -> Second Order Linear Actuator2/1
  Data Type Conversion8/1 -> Second Order Linear Actuator1/1
  Data Type Conversion7/1 -> Second Order Linear Actuator/1
  Rate Transition3/1 -> [dtAct]
  Rate Transition2/1 -> [drAct]
  Rate Transition1/1 -> [daAct]
  Second Order Linear Actuator4/1 -> Angle Conversion3/1
  Second Order Linear Actuator3/1 -> Rate Transition3/1, "dt "/1
  Second Order Linear Actuator2/1 -> Angle Conversion2/1
  Second Order Linear Actuator1/1 -> Angle Conversion1/1
  Second Order Linear Actuator/1 -> Angle Conversion/1
  "df, rad"/1 -> Data Type Conversion11/1
  dt/1 -> Data Type Conversion10/1
  "dr, rad"/1 -> Data Type Conversion9/1
  da,rad/1 -> Data Type Conversion8/1
  de,rad/1 -> Data Type Conversion7/1

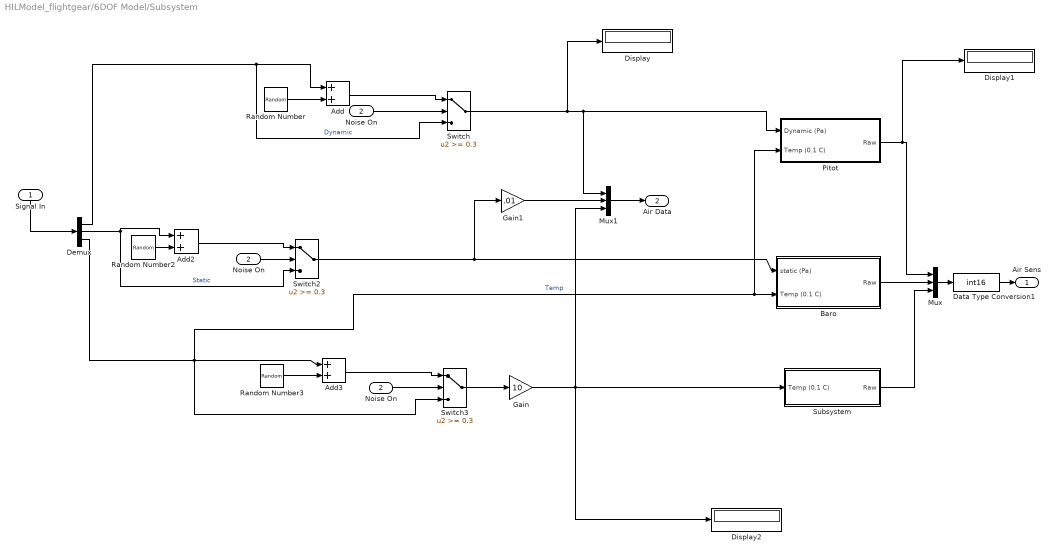
== system HILModel_flightgear/6DOF Model/Subsystem ==
  Signal In : Inport
  Noise On : Inport  Port=2
  Add : Sum
  Add2 : Sum
  Add3 : Sum
  Baro : Subsystem
  Data Type Conversion1 : DataTypeConversion  OutDataTypeStr=int16
  Demux : Demux  Outputs=3
  Display : Display
  Display1 : Display
  Display2 : Display
  Gain : Gain  Gain=10
  Gain1 : Gain  Gain=.01
  Mux : Mux  Inputs=3
  Mux1 : Mux  Inputs=3
  "Noise On " : InportShadow  Port=2
  "Noise On  " : InportShadow  Port=2
  Pitot : Subsystem
  Random Number : RandomNumber  Variance=nv(1)  Seed=ns(1)  SampleTime=st
  Random Number2 : RandomNumber  Variance=nv(2)  Seed=ns(2)  SampleTime=st
  Random Number3 : RandomNumber  Variance=nv(3)  Seed=ns(3)  SampleTime=st
  Subsystem : Subsystem
  Switch : Switch  Threshold=0.3
  Switch2 : Switch  Threshold=0.3
  Switch3 : Switch  Threshold=0.3
  Air Sens : Outport
  Air Data : Outport  Port=2
  wires:
  Noise On/1 -> Switch/2
  Add/1 -> Switch/1
  Random Number/1 -> Add/2
  Mux/1 -> Data Type Conversion1/1
  Add2/1 -> Switch2/1
  Random Number2/1 -> Add2/2
  "Noise On  "/1 -> Switch3/2
  Add3/1 -> Switch3/1
  Random Number3/1 -> Add3/2
  Subsystem/1(Raw) -> Mux/3
  Signal In/1 -> Demux/1
  Demux/3 -> Add3/1, Switch3/3, Baro/2(Temp (0.1 C)), Pitot/2(Temp (0.1 C))  "Temp"
  "Noise On "/1 -> Switch2/2
  Demux/2 -> Add2/1, Switch2/3  "Static"
  Baro/1(Raw) -> Mux/2
  Switch2/1 -> Baro/1(static (Pa)), Gain1/1
  Switch3/1 -> Gain/1
  Switch/1 -> Pitot/1(Dynamic (Pa)), Mux1/1, Display/1
  Data Type Conversion1/1 -> Air Sens/1
  Pitot/1(Raw) -> Mux/1, Display1/1
  Mux1/1 -> Air Data/1
  Demux/1 -> Add/1, Switch/3  "Dynamic"
  Gain/1 -> Subsystem/1(Temp (0.1 C)), Mux1/3, Display2/1
  Gain1/1 -> Mux1/2

== system HILModel_flightgear/6DOF Model/Subsystem2 ==
  Signal In : Inport
  Noise On : Inport  Port=2
  Add : Sum
  Data Type Conversion4 : DataTypeConversion  OutDataTypeStr=single
  Random Number : RandomNumber  Variance=nv  Seed=ns  SampleTime=st
  Signal1 : InportShadow  Port=1
  Switch : Switch  Threshold=0.3
  Signal Out : Outport
  wires:
  Signal1/1 -> Switch/3
  Switch/1 -> Data Type Conversion4/1
  Noise On/1 -> Switch/2
  Signal In/1 -> Add/1
  Add/1 -> Switch/1
  Random Number/1 -> Add/2
  Data Type Conversion4/1 -> Signal Out/1

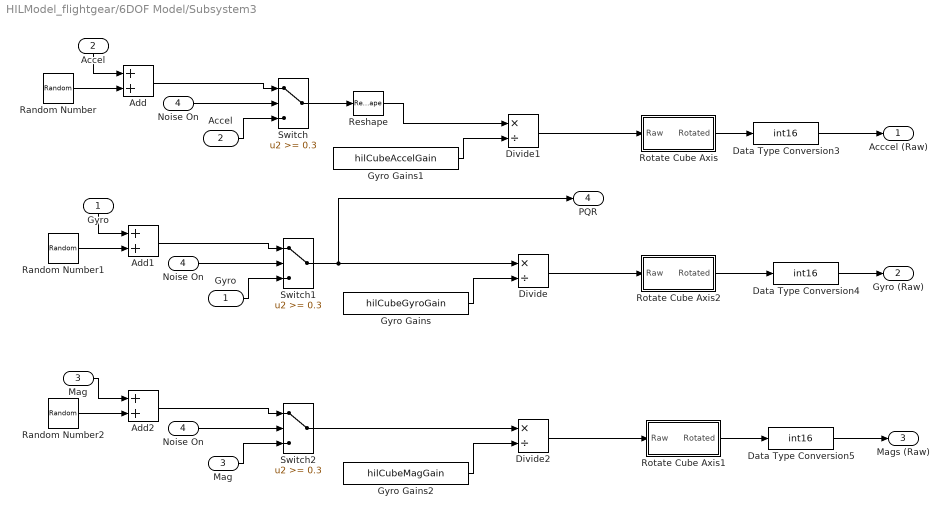
== system HILModel_flightgear/6DOF Model/Subsystem3 ==
  Gyro : Inport
  Accel : Inport  Port=2
  Mag : Inport  Port=3
  Noise On : Inport  Port=4
  "Accel " : InportShadow  Port=2
  Add : Sum
  Add1 : Sum
  Add2 : Sum
  Data Type Conversion3 : DataTypeConversion  OutDataTypeStr=int16
  Data Type Conversion4 : DataTypeConversion  OutDataTypeStr=int16
  Data Type Conversion5 : DataTypeConversion  OutDataTypeStr=int16
  Divide : Product  Inputs=*/  OutDataTypeStr=single
  Divide1 : Product  Inputs=*/  OutDataTypeStr=single
  Divide2 : Product  Inputs=*/  OutDataTypeStr=single
  "Gyro " : InportShadow  Port=1
  Gyro Gains : Constant  Value=hilCubeGyroGain  OutDataTypeStr=single
  Gyro Gains1 : Constant  Value=hilCubeAccelGain  OutDataTypeStr=single
  Gyro Gains2 : Constant  Value=hilCubeMagGain  OutDataTypeStr=single
  "Mag " : InportShadow  Port=3
  "Noise On " : InportShadow  Port=4
  "Noise On  " : InportShadow  Port=4
  Random Number : RandomNumber  Variance=accelVar  Seed=accelSeed  SampleTime=st
  Random Number1 : RandomNumber  Variance=gyroVar  Seed=gyroSeed  SampleTime=st
  Random Number2 : RandomNumber  Variance=magVar  Seed=magSeed  SampleTime=st
  Reshape : Reshape
  Rotate Cube Axis : Subsystem
  Rotate Cube Axis1 : Subsystem
  Rotate Cube Axis2 : Subsystem
  Switch : Switch  Threshold=0.3
  Switch1 : Switch  Threshold=0.3
  Switch2 : Switch  Threshold=0.3
  Acccel (Raw) : Outport
  "Gyro (Raw)  " : Outport  Port=2
  Mags (Raw) : Outport  Port=3
  "PQR " : Outport  Port=4
  wires:
  Random Number/1 -> Add/2
  Add/1 -> Switch/1
  Accel/1 -> Add/1
  Noise On/1 -> Switch/2
  "Accel "/1 -> Switch/3
  Random Number1/1 -> Add1/2
  Add1/1 -> Switch1/1
  Gyro/1 -> Add1/1
  "Noise On "/1 -> Switch1/2
  "Gyro "/1 -> Switch1/3
  Gyro Gains/1 -> Divide/2
  Switch1/1 -> "PQR "/1, Divide/1
  Switch/1 -> Reshape/1
  Gyro Gains1/1 -> Divide1/2
  Random Number2/1 -> Add2/2
  Add2/1 -> Switch2/1
  "Mag "/1 -> Add2/1
  "Noise On  "/1 -> Switch2/2
  Mag/1 -> Switch2/3
  Gyro Gains2/1 -> Divide2/2
  Switch2/1 -> Divide2/1
  Divide1/1 -> Rotate Cube Axis/1(Raw)
  Divide/1 -> Rotate Cube Axis2/1(Raw)
  Divide2/1 -> Rotate Cube Axis1/1(Raw)
  Rotate Cube Axis/1(Rotated) -> Data Type Conversion3/1
  Rotate Cube Axis2/1(Rotated) -> Data Type Conversion4/1
  Rotate Cube Axis1/1(Rotated) -> Data Type Conversion5/1
  Reshape/1 -> Divide1/1
  Data Type Conversion3/1 -> Acccel (Raw)/1
  Data Type Conversion4/1 -> "Gyro (Raw)  "/1
  Data Type Conversion5/1 -> Mags (Raw)/1

== system HILModel_flightgear/6DOF Model/Subsystem5 ==
  Signal In : Inport
  Noise On : Inport  Port=2
  Add : Sum
  Data Type Conversion4 : DataTypeConversion  OutDataTypeStr=single
  Random Number : RandomNumber  Variance=nv  Seed=ns  SampleTime=st
  Signal1 : InportShadow  Port=1
  Switch : Switch  Threshold=0.3
  Signal Out : Outport
  wires:
  Signal1/1 -> Switch/3
  Switch/1 -> Data Type Conversion4/1
  Noise On/1 -> Switch/2
  Signal In/1 -> Add/1
  Add/1 -> Switch/1
  Random Number/1 -> Add/2
  Data Type Conversion4/1 -> Signal Out/1

== system HILModel_flightgear/6DOF Model/Subsystem6 ==
  Signal In : Inport
  Noise On : Inport  Port=2
  Add : Sum
  Data Type Conversion4 : DataTypeConversion  OutDataTypeStr=single
  Random Number : RandomNumber  Variance=nv  Seed=ns  SampleTime=st
  Signal1 : InportShadow  Port=1
  Switch : Switch  Threshold=0.3
  Signal Out : Outport
  wires:
  Random Number/1 -> Add/2
  Add/1 -> Switch/1
  Signal In/1 -> Add/1
  Noise On/1 -> Switch/2
  Switch/1 -> Data Type Conversion4/1
  Signal1/1 -> Switch/3
  Data Type Conversion4/1 -> Signal Out/1

== system HILModel_flightgear/From AP/Subsystem ==
  uS : Inport
  Data Type Conversion : DataTypeConversion  OutDataTypeStr=uint16
  Gain : Gain  Gain=2.5
  PWM : Outport
  wires:
  Gain/1 -> Data Type Conversion/1
  Data Type Conversion/1 -> PWM/1
  uS/1 -> Gain/1

== system HILModel_flightgear/From AP/Subsystem1 ==
  uS : Inport
  Data Type Conversion : DataTypeConversion  OutDataTypeStr=uint16
  Gain : Gain  Gain=2.5
  PWM : Outport
  wires:
  uS/1 -> Gain/1
  Data Type Conversion/1 -> PWM/1
  Gain/1 -> Data Type Conversion/1

== system HILModel_flightgear/From AP/Subsystem2 ==
  uS : Inport
  Data Type Conversion : DataTypeConversion  OutDataTypeStr=uint16
  Gain : Gain  Gain=2.5
  PWM : Outport
  wires:
  Gain/1 -> Data Type Conversion/1
  Data Type Conversion/1 -> PWM/1
  uS/1 -> Gain/1

== system HILModel_flightgear/From AP/Subsystem3 ==
  uS : Inport
  Data Type Conversion : DataTypeConversion  OutDataTypeStr=uint16
  Gain : Gain  Gain=2.5
  PWM : Outport
  wires:
  uS/1 -> Gain/1
  Data Type Conversion/1 -> PWM/1
  Gain/1 -> Data Type Conversion/1

== system HILModel_flightgear/Get Delay/Detect Change ==
  Data : Inport
  Abs1 : Abs  SampleTime=SampleT
  Difference1 : simulink/Discrete/Difference  ICPrevInput=0.0  InputProcessing=Inherited  OutMin=[]  OutMax=[]  OutDataType=sfix(16)  OutScaling=2^-10  DoSatur=off
  Saturation1 : Saturate  UpperLimit=1  LowerLimit=0  SampleTime=SampleT
  change? : Outport
  wires:
  Difference1/1 -> Abs1/1
  Abs1/1 -> Saturation1/1
  Data/1 -> Difference1/1
  Saturation1/1 -> change?/1

== system HILModel_flightgear/Get Delay/GPSAlive ==
  update? : Inport
  Constant : Constant
  Constant1 : Constant  Value=0
  Constant2 : Constant  Value=SampleT
  Discrete-Time Integrator : DiscreteIntegrator  ExternalReset=rising  InitialConditionSource=external  SampleTime=SampleT  ICPrevOutput=DiscIntNeverNeededParam  ICPrevScaledInput=DiscIntNeverNeededParam
  Integer Delay2 : Delay  DelayLength=1  InputProcessing=Inherited
  Sum : Sum  Inputs=|++
  Update TIme : Outport
  wires:
  Constant/1 -> Discrete-Time Integrator/1
  Constant1/1 -> Discrete-Time Integrator/3
  Discrete-Time Integrator/1 -> Integer Delay2/1
  update?/1 -> Discrete-Time Integrator/2
  Integer Delay2/1 -> Sum/1
  Constant2/1 -> Sum/2
  Sum/1 -> Update TIme/1

== system HILModel_flightgear/6DOF Model/Plant/6-DOF EOM ==
  "[F,M]" : Inport
  Vb Corr : Inport  Port=2
  Angular Rates : Integrator  InitialCondition=PQR_0'
  Demux1 : Demux  Outputs=2
  Euler Angles : Integrator  InitialCondition=Euler_0
  Get Euler Dot : Subsystem
      mask Display:
      | port_label('input', 1, 'p, q, r')
      | port_label('input', 2, 'Euler')
      | port_label('output', 1, 'Euler_dot')
  Mux : Mux  Inputs=[3;3]
  NED2NEU : Gain  Gain=[1 0 0;0 1 0;0 0 -1]  Multiplication=Matrix(K*u)  SaturateOnIntegerOverflow=on  OutDataTypeStr=Inherit: Same as input  ParamDataTypeStr=Inherit: Same as input
  Position : Integrator  InitialCondition=Pos_0'
  RB2L * Vb : Product  Multiplication=Matrix(*)  SaturateOnIntegerOverflow=on  InputSameDT=on  OutDataTypeStr=Inherit: Same as first input
  RB2LTP : Subsystem
  Velocities Body : Integrator  InitialCondition=Vb_0'
  "[V1,2,3,W1,2,3]" : Subsystem
  X,Y,Z (LTP) : Outport
  "Vx, Vy, Vz" : Outport  Port=2
  Euler : Outport  Port=3
  "p, q, r" : Outport  Port=4
  Vb : Outport  Port=5
  Ab meas : Outport  Port=6
  Euler_dot : Outport  Port=7
  wires:
  "[V1,2,3,W1,2,3]"/1("Acc_meas ") -> Ab meas/1
  Euler Angles/1 -> "[V1,2,3,W1,2,3]"/2(Euler), Get Euler Dot/2(Euler), Euler/1, RB2LTP/1(Euler)
  Demux1/1 -> Velocities Body/1
  "[V1,2,3,W1,2,3]"/2(V*dot) -> Demux1/1
  Demux1/2 -> Angular Rates/1
  "[F,M]"/1 -> "[V1,2,3,W1,2,3]"/1("[F ; M]")
  RB2LTP/1(Rot) -> RB2L * Vb/1
  Velocities Body/1 -> Vb/1, RB2L * Vb/2
  Mux/1 -> "[V1,2,3,W1,2,3]"/3(V*)
  Position/1 -> X,Y,Z (LTP)/1
  Angular Rates/1 -> Get Euler Dot/1(p,q,r), Mux/2, "p, q, r"/1
  RB2L * Vb/1 -> NED2NEU/1, "Vx, Vy, Vz"/1  "NED"
  NED2NEU/1 -> Position/1
  Get Euler Dot/1(Euler_dot) -> Euler Angles/1, Euler_dot/1
  Vb Corr/1 -> Mux/1

== system HILModel_flightgear/6DOF Model/Plant/Engine Model ==
  dt : Inport
  Vmag : Inport  Port=2
  Constant4 : Constant  Value=0
  Get To1 : Subsystem
  Mux : Mux  Inputs=2
  Mux1 : Mux  Inputs=3
  Thrust Available (lbs) : Fcn  Expr=u(1) - 0.047*sqrt(u(1))*u(2)
  kg2N : Gain  Gain=ISA_g  SaturateOnIntegerOverflow=on  OutDataTypeStr=Inherit: Same as input  ParamDataTypeStr=Inherit: Same as input
  lbs2kg : Gain  Gain=0.45359237  SaturateOnIntegerOverflow=on  OutDataTypeStr=Inherit: Same as input  ParamDataTypeStr=Inherit: Same as input
  Thrust : Outport
  wires:
  dt/1 -> Get To1/1(dt)
  Get To1/1(To) -> Mux/1
  Mux/1 -> Thrust Available (lbs)/1
  Thrust Available (lbs)/1 -> lbs2kg/1
  Vmag/1 -> Mux/2
  Mux1/1 -> Thrust/1
  lbs2kg/1 -> kg2N/1
  Constant4/1 -> Mux1/2, Mux1/3
  kg2N/1 -> Mux1/1

== system HILModel_flightgear/6DOF Model/Plant/Forces and Moments ==
  "Wind {E}" : Inport
  Rho : Inport  Port=2
  "de, deg" : Inport  Port=3
  daL,deg : Inport  Port=4
  daR,deg : Inport  Port=5
  "dr, deg" : Inport  Port=6
  "df, deg" : Inport  Port=7
  "Vx, Vy, Vz " : Inport  Port=8
  Euler : Inport  Port=9  PortDimensions=3
  p,q,r : Inport  Port=10
  Alpha/Beta : Subsystem
  Body Frame F & M : Subsystem
  Get Grav Force in Body : Subsystem
  Gravitational Force : Constant  Value=[0 0 mass*ISA_g]  VectorParams1D=off
  NED(u)2b : Subsystem
  Sum : Sum  Inputs=|++  SaturateOnIntegerOverflow=on
  Vair : Sum  Inputs=+-  SaturateOnIntegerOverflow=on  InputSameDT=on  OutDataTypeStr=Inherit: Same as first input
  Airspeed : Outport
  Forces : Outport  Port=2
  Moments : Outport  Port=3
  Vb Corr : Outport  Port=4
  q (Pa) : Outport  Port=5
  wires:
  Get Grav Force in Body/1(Grav Force (Body)) -> Sum/2
  Alpha/Beta/5(q (Pa)) -> q (Pa)/1
  "Vx, Vy, Vz "/1 -> Vair/1
  Vair/1 -> NED(u)2b/1(V w)
  Euler/1 -> NED(u)2b/2(Euler), Get Grav Force in Body/1(Euler)
  Rho/1 -> Alpha/Beta/2(Rho)
  NED(u)2b/1(Vb Corr) -> Alpha/Beta/1("Vx, Vy, Vz (Body)"), Vb Corr/1
  Body Frame F & M/2(M_b) -> Moments/1
  Gravitational Force/1 -> Get Grav Force in Body/2(Grav Force)
  Body Frame F & M/1(F_b) -> Sum/1
  Sum/1 -> Forces/1
  Alpha/Beta/3(qS) -> Body Frame F & M/3(qs)
  Alpha/Beta/4(Speed) -> Body Frame F & M/4(Airspeed), Airspeed/1
  "df, deg"/1 -> Body Frame F & M/9("df, deg")
  p,q,r/1 -> Body Frame F & M/10(p,q,r)
  Alpha/Beta/2("beta, deg") -> Body Frame F & M/2("Beta, deg")
  "dr, deg"/1 -> Body Frame F & M/8("dr, deg")
  daL,deg/1 -> Body Frame F & M/6("daL, deg")
  Alpha/Beta/1("alpha, deg") -> Body Frame F & M/1("Alpha, deg")
  "de, deg"/1 -> Body Frame F & M/5("de, deg")
  "Wind {E}"/1 -> Vair/2
  daR,deg/1 -> Body Frame F & M/7("daR, deg")

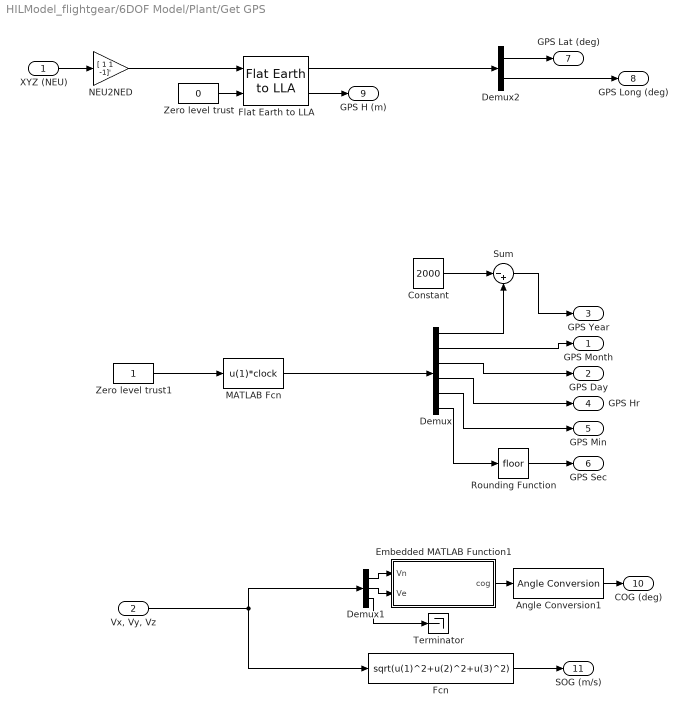
== system HILModel_flightgear/6DOF Model/Plant/Get GPS ==
  XYZ (NEU) : Inport
  "Vx, Vy, Vz" : Inport  Port=2
  Angle Conversion1 : aerolibconvert2/Angle Conversion  IU=rad  OU=deg
  Constant : Constant  Value=2000
  Demux : Demux  Outputs=6
  Demux1 : Demux  Outputs=3
  Demux2 : Demux  Outputs=2
  Embedded MATLAB Function1 : MATLAB Function  TreatAsAtomicUnit=on
  Fcn : Fcn  Expr=sqrt(u(1)^2+u(2)^2+u(3)^2)
  Flat Earth to LLA : aerolibtransform2/Flat Earth to LLA  units=Metric (MKS)  ptype=Earth (WGS84)  F=1/298.257223563  R=6378137  LL0=[GS_location(2) GS_location(3)]  psi=0
  MATLAB Fcn : MATLABFcn  MATLABFcn=u(1)*clock  OutputSignalType=real  SampleTime=SampleT
  NEU2NED : Gain  Gain=[ 1 1 -1]'  SaturateOnIntegerOverflow=on  OutDataTypeStr=Inherit: Same as input  ParamDataTypeStr=Inherit: Same as input
  Rounding Function : Rounding
  Sum : Sum  Inputs=|-+
  Terminator : Terminator
  Zero level trust : Constant  Value=0  SampleTime=SampleT
  Zero level trust1 : Constant  SampleTime=SampleT
  GPS Month : Outport
  GPS Day : Outport  Port=2
  GPS Year : Outport  Port=3
  GPS Hr : Outport  Port=4
  GPS Min : Outport  Port=5
  GPS Sec : Outport  Port=6
  GPS Lat (deg) : Outport  Port=7
  GPS Long (deg) : Outport  Port=8
  GPS H (m) : Outport  Port=9
  COG (deg) : Outport  Port=10
  SOG (m/s) : Outport  Port=11
  wires:
  NEU2NED/1 -> Flat Earth to LLA/1
  Zero level trust/1 -> Flat Earth to LLA/2
  XYZ (NEU)/1 -> NEU2NED/1
  Flat Earth to LLA/1 -> Demux2/1
  Flat Earth to LLA/2 -> GPS H (m)/1
  Zero level trust1/1 -> MATLAB Fcn/1
  MATLAB Fcn/1 -> Demux/1
  Demux/2 -> GPS Month/1
  Demux/3 -> GPS Day/1
  Demux/4 -> GPS Hr/1
  Demux/5 -> GPS Min/1
  Demux/6 -> Rounding Function/1
  Rounding Function/1 -> GPS Sec/1
  Demux2/1 -> GPS Lat (deg)/1
  Demux2/2 -> GPS Long (deg)/1
  Fcn/1 -> SOG (m/s)/1
  Demux1/1 -> Embedded MATLAB Function1/1(Vn)
  Demux1/2 -> Embedded MATLAB Function1/2(Ve)
  "Vx, Vy, Vz"/1 -> Demux1/1, Fcn/1
  Embedded MATLAB Function1/1(cog) -> Angle Conversion1/1
  Angle Conversion1/1 -> COG (deg)/1
  Demux/1 -> Sum/2
  Constant/1 -> Sum/1
  Sum/1 -> GPS Year/1
  Demux1/3 -> Terminator/1
